simulink model "Metal_hydride_tank_Model_charge_Keow"  (R2022b)
settings: Solver=FixedStepAuto  StartTime=0.0  StopTime=54000  FixedStep=5e-3  MaxStep=0.005  RelTol=1e-3
values from neighbouring files (symbols this model uses):
  a = 13.7    [Metal_hydride_tank_Model_charge_Keow_run.m]
  A_s = 1.347    [Metal_hydride_tank_Model_charge_Keow_run.m]
  b = 3704    [Metal_hydride_tank_Model_charge_Keow_run.m]
  beta = 0.11414    [Metal_hydride_tank_Model_charge_Keow_run.m]
  C_a = 59.187    [Metal_hydride_tank_Model_charge_Keow_run.m]
  C_d = 9.57    [Metal_hydride_tank_Model_charge_Keow_run.m]
  C_pg = 14890    [Metal_hydride_tank_Model_charge_Keow_run.m]
  C_ps = 419    [Metal_hydride_tank_Model_charge_Keow_run.m]
  C_pw = 1860    [Metal_hydride_tank_Model_charge_Keow_run.m]
  Delta_Ha = 30478    [Metal_hydride_tank_Model_charge_Keow_run.m]
  Delta_Hd = 30800    [Metal_hydride_tank_Model_charge_Keow_run.m]
  E_a = 21179.6    [Metal_hydride_tank_Model_charge_Keow_run.m]
  E_d = 16420    [Metal_hydride_tank_Model_charge_Keow_run.m]
  epsilon = 0.5    [Metal_hydride_tank_Model_charge_Keow_run.m]
  f_w = 0.1667    [Metal_hydride_tank_Model_charge_Keow_run.m]
  m_MH = 47    [Metal_hydride_tank_Model_charge_Keow_run.m]
  MW_H2 = 2.01598e-3    (= 0.00201598)    [Metal_hydride_tank_Model_charge_Keow_run.m]
  P_0 = 101325    [Metal_hydride_tank_Model_charge_Keow_run.m]
  P_ref = 1500000    [Metal_hydride_tank_Model_charge_Keow_run.m]
  Phi = 0.33    [Metal_hydride_tank_Model_charge_Keow_run.m]
  Phi_0 = 0.008584    [Metal_hydride_tank_Model_charge_Keow_run.m]
  R_u = 8.314472    [Metal_hydride_tank_Model_charge_Keow_run.m]
  rho_H2 = 0.0897    [Metal_hydride_tank_Model_charge_Keow_run.m]
  rho_s0 = 8400    [Metal_hydride_tank_Model_charge_Keow_run.m]
  T_win = 293.15    [Metal_hydride_tank_Model_charge_Keow_run.m]
  U = 25    [Metal_hydride_tank_Model_charge_Keow_run.m]
  V_H2 = 7.849    [Metal_hydride_tank_Model_charge_Keow_run.m]
  V_tank = 0.0165    [Metal_hydride_tank_Model_charge_Keow_run.m]
settings Model: Creator=76593  LastModifiedBy=cmingrui
settings SolverCC: AlgebraicLoopSolver=TrustRegion
settings DataIOCC: ReturnWorkspaceOutputs=off
settings DebuggingCC: UnconnectedInputMsg=warning  UnconnectedOutputMsg=warning  UnconnectedLineMsg=warning  SFMachineParentedDataDiag=warning
settings ModelReferenceCC: EnableRefExpFcnMdlSchedulingChecks=on
settings RTWCC: DLArmComputeVersion=19.05

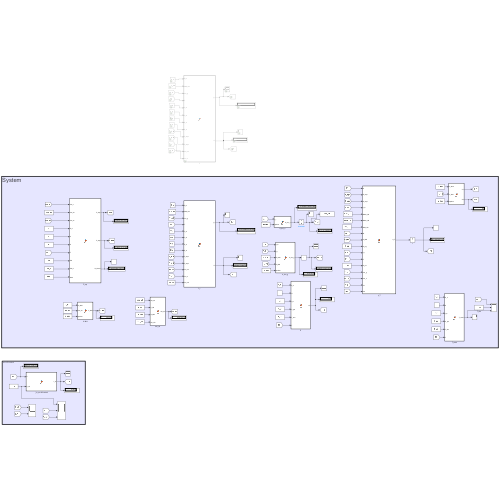
[thumbnail: Simulink's stored preview of the top-level diagram]
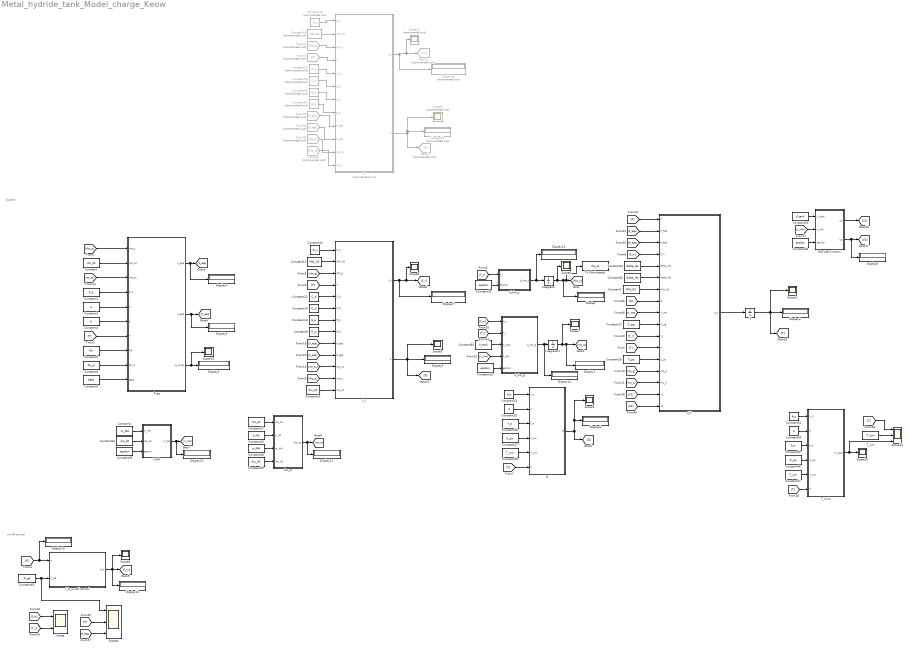
== system Metal_hydride_tank_Model_charge_Keow ==
  note: on-off control
  note: System
  1 : MATLAB Function  Commented=on  TreatAsAtomicUnit=on
  Constant{,24,31,37} (4 alike) : Constant  Value=rho_s0
  Constant1 : Constant  Value=m_MH
  Constant10 : Constant  Value=R_u
  Constant11 : Constant  Value=MW_H2
  Constant12 : Constant  Value=C_a
  Constant13 : Constant  Value=E_a
  Constant14 : Constant  Value=C_d
  Constant15 : Constant  Commented=on  Value=R_u
  Constant16 : Constant  Commented=on  Value=MW_H2
  Constant17 : Constant  Value=C_pg
  Constant{18..19,35..36} (4 alike) : Constant  Value=epsilon
  Constant2 : Constant  Value=P_0
  Constant20 : Constant  Value=C_ps
  Constant21 : Constant  Value=Delta_Ha
  Constant22 : Constant  Commented=on  Value=C_a
  Constant23 : Constant  Value=A_s
  Constant25 : Constant  Value=U
  Constant26 : Constant  Value=f_w
  Constant27 : Constant  Value=C_pw
  Constant28 : Constant  Value=T_win
  Constant29 : Constant  Value=V_tank
  Constant3 : Constant  Value=a
  Constant30 : Constant  Value=V_tank
  Constant32 : Constant  Value=Delta_Hd
  Constant33 : Constant  Commented=on  Value=E_a
  Constant34 : Constant  Commented=on  Value=C_d
  Constant38 : Constant  Value=m_MH
  Constant39 : Constant  Value=rho_H2
  Constant4 : Constant  Value=b
  Constant41 : Constant  Commented=on  Value=E_d
  Constant43 : Constant  Value=V_H2
  Constant47 : Constant  Value=T_win
  Constant48 : Constant  Value=C_pw
  Constant49 : Constant  Value=f_w
  Constant5 : Constant  Value=Phi
  Constant50 : Constant  Value=U
  Constant51 : Constant  Value=A_s
  Constant6 : Constant  Value=Phi_0
  Constant65 : Constant  Value=P_ref
  Constant7 : Constant  Value=MW_H2
  Constant8 : Constant  Value=E_d
  Constant9 : Constant  Value=beta
  Display{,1..14,19} (16 alike) : Display
  Display15 : Display  Commented=on
  Display16 : Display  Commented=on
  From26 : From  Commented=on  GotoTag=rho_ss
  From29 : From  Commented=on  GotoTag=P_eqa
  From30 : From  Commented=on  GotoTag=P_eqd
  From31 : From  Commented=on  GotoTag=rho_g
  From32 : From  Commented=on  GotoTag=rho_s
  From33 : From  Commented=on  GotoTag=T
  Goto11 : Goto  Commented=on  GotoTag=f_r
  Goto5 : Goto  Commented=on  GotoTag=P
  Integrator : Integrator  InitialCondition=8412.4
  Integrator1 : Integrator  InitialCondition=0.0831
  MATLAB Function : MATLAB Function  TreatAsAtomicUnit=on
  P_eq : MATLAB Function  TreatAsAtomicUnit=on
  Q : MATLAB Function  TreatAsAtomicUnit=on
  Scope : Scope  NumInputPorts=2
  Scope{1..3,6..10,15} (9 alike) : Scope
  Scope11 : Scope  NumInputPorts=3
  Scope12 : Scope  Commented=on
  Scope4 : Scope  NumInputPorts=3
  Scope5 : Scope  Commented=on
  T : Integrator  InitialCondition=293.15
  T_win : Constant  Value=T_win
  T_wout : MATLAB Function  TreatAsAtomicUnit=on
  To Workspace1 : ToWorkspace  VariableName=rho_s1  SampleTime=-1
  V_MH : MATLAB Function  TreatAsAtomicUnit=on
  d_T : MATLAB Function  TreatAsAtomicUnit=on
  d_rho_g : MATLAB Function  TreatAsAtomicUnit=on
  d_rho_s : MATLAB Function  TreatAsAtomicUnit=on
  f_in_on-off control : MATLAB Function  TreatAsAtomicUnit=on
  f_r : MATLAB Function  TreatAsAtomicUnit=on
  rho_ss : MATLAB Function  TreatAsAtomicUnit=on
  wires:
  Integrator/1 -> Scope6/1, Display/1, To Workspace1/1, [rho_s]
  d_rho_g/1(d_rho_g) -> Display14/1, Integrator1/1
  Integrator1/1 -> Scope7/1, Display1/1, [rho_g]
  d_T/1(d_T) -> T/1
  [T] -> d_T/12(T)
  [rho_s] -> P_eq/1(rho_s)
  Constant/1 -> P_eq/2(rho_s0)
  [rho_ss] -> P_eq/3(rho_ss)
  Constant2/1 -> P_eq/4(P_0)
  Constant3/1 -> P_eq/5(a)
  Constant4/1 -> P_eq/6(b)
  [T] -> P_eq/7(T)
  Constant5/1 -> P_eq/8(Phi)
  Constant6/1 -> P_eq/9(Phi_0)
  Constant9/1 -> P_eq/10(beta)
  Constant10/1 -> f_r/1(R_u)
  [T] -> f_r/4(T)
  Constant12/1 -> f_r/5(C_a)
  Constant13/1 -> f_r/7(E_a)
  [rho_ss] -> f_r/11(rho_ss)
  Constant17/1 -> d_T/10(C_pg)
  Constant19/1 -> d_rho_g/5(epsilon)
  Constant20/1 -> d_T/13(C_ps)
  Q/1(Q) -> [Q], Scope1/1, Display6/1
  [T] -> Q/6(T)
  Constant23/1 -> Q/1(A_s)
  Constant25/1 -> Q/2(U)
  Constant26/1 -> Q/3(f_w)
  Constant27/1 -> Q/4(C_pw)
  Constant28/1 -> Q/5(T_win)
  Constant30/1 -> d_rho_g/3(V_tank)
  [V_MH] -> d_rho_g/4(V_MH)
  f_r/2(P) -> Scope3/1, Display3/1, [P]
  Constant35/1 -> d_rho_s/2(epsilon)
  T/1 -> [T], Scope2/1, Display2/1
  P_eq/3(H_Hmax) -> Scope15/1, Display5/1
  [f_in] -> d_T/4(f_in)
  [rho_g] -> d_T/14(rho_g)
  [rho_s] -> d_T/15(rho_s)
  [f_in] -> d_rho_g/1(f_in)
  [f_r] -> d_rho_g/2(f_r)
  V_MH/1(V_MH) -> Display10/1, [V_MH]
  Constant24/1 -> V_MH/2(rho_s0)
  Constant36/1 -> V_MH/3(epsilon)
  Constant37/1 -> rho_ss/1(rho_s0)
  rho_ss/1(rho_ss) -> Display11/1, [rho_ss]
  Constant43/1 -> rho_ss/2(V_H2)
  Constant38/1 -> rho_ss/3(m_MH)
  Constant39/1 -> rho_ss/4(rho_H2)
  Constant1/1 -> V_MH/1(m_MH)
  Constant7/1 -> d_T/7(MW_H2)
  Constant8/1 -> f_r/8(E_d)
  Constant14/1 -> f_r/6(C_d)
  Constant31/1 -> f_r/13(rho_s0)
  P_eq/1(P_eqa) -> Display4/1, [P_eqa]
  P_eq/2(P_eqd) -> Display9/1, [P_eqd]
  [P_eqa] -> f_r/9(P_eqa)
  [P_eqd] -> f_r/10(P_eqd)
  [f_r] -> d_T/11(f_r)
  Constant21/1 -> d_T/5(Delta_Ha)
  Constant32/1 -> d_T/6(Delta_Hd)
  [P] -> d_T/1(P)
  [P_eqa] -> d_T/2(P_eqa)
  [rho_s] -> f_r/12(rho_s)
  [rho_g] -> f_r/3(rho_g)
  [P] -> Display19/1, f_in_on-off control/1(P)
  f_in_on-off control/1(f_in) -> Scope8/1, [f_in], Display12/1
  [f_in] -> Scope/1
  [f_r] -> Scope/2
  [P] -> Scope4/2
  Constant65/1 -> f_in_on-off control/2(P_ref), Scope4/1
  [P_eqa] -> Scope4/3
  [T] -> T_wout/6(T)
  Constant47/1 -> T_wout/5(T_win)
  Constant48/1 -> T_wout/4(C_pw)
  Constant49/1 -> T_wout/3(f_w)
  Constant50/1 -> T_wout/2(U)
  Constant51/1 -> T_wout/1(A_s)
  T_wout/1(T_wout) -> Scope11/3, Scope10/1
  [P_eqd] -> d_T/3(P_eqd)
  T_win/1 -> Scope11/2
  d_rho_s/1(d_rho_s) -> Integrator/1, Display13/1
  f_r/1(f_r) -> Display7/1, Scope9/1, [f_r]
  [f_r] -> d_rho_s/1(f_r)
  Constant11/1 -> f_r/2(MW_H2)
  [Q] -> d_T/8(Q)
  [V_MH] -> d_T/9(V_MH)
  MATLAB Function/1(V1) -> [V1]
  MATLAB Function/2(V2) -> Display8/1, [V2]
  Constant29/1 -> MATLAB Function/1(V_tank)
  [V_MH] -> MATLAB Function/2(V_MH)
  Constant18/1 -> MATLAB Function/3(epsilon)
  [T] -> Scope11/1
  [V1] -> d_T/16(V1)
  [V2] -> d_T/17(V2)
  Constant16/1 -> 1/2(MW_H2)
  1/1(f_r) -> Goto11/1, Scope12/1, Display16/1
  From31/1 -> 1/3(rho_g)
  From32/1 -> 1/12(rho_s)
  From30/1 -> 1/10(P_eqd)
  From29/1 -> 1/9(P_eqa)
  Constant34/1 -> 1/6(C_d)
  Constant41/1 -> 1/8(E_d)
  1/2(P) -> Display15/1, Scope5/1, Goto5/1
  From26/1 -> 1/11(rho_ss)
  Constant33/1 -> 1/7(E_a)
  Constant22/1 -> 1/5(C_a)
  From33/1 -> 1/4(T)
  Constant15/1 -> 1/1(R_u)

== matlab function Metal_hydride_tank_Model_charge_Keow/d_rho_g ==
  data: f_in input; f_r input; V_tank input; V_MH input; d_rho_g output; epsilon input
function d_rho_g = fcn(f_in,f_r,V_tank,V_MH,epsilon)

V1=V_tank/V_MH-1+epsilon;
d_rho_g = (f_in-f_r)/V1;

== matlab function Metal_hydride_tank_Model_charge_Keow/d_T ==
  data: P input; P_eqa input; P_eqd input; f_in input; Delta_Ha input; Delta_Hd input; MW_H2 input; Q input; V_MH input; C_pg input; d_T output; f_r input; T input; C_ps input; rho_g input; rho_s input; V1 input; V2 input
 function d_T  = fcn(P,P_eqa,P_eqd,f_in,Delta_Ha,Delta_Hd,MW_H2,Q,V_MH,C_pg,f_r,T,C_ps,rho_g,rho_s,V1,V2)

if P>P_eqa
    d_T = (-C_pg*(f_in-f_r)*T-C_ps*f_r*T+f_r*Delta_Ha/MW_H2+Q/V_MH)/(V1*C_pg*rho_g+V2*C_ps*rho_s);
elseif P<P_eqd
    d_T = (-C_pg*(f_in-f_r)*T-C_ps*f_r*T+f_r*Delta_Hd/MW_H2+Q/V_MH)/(V1*C_pg*rho_g+V2*C_ps*rho_s);
else
    d_T = (-C_pg*f_in*T+Q/V_MH)/(V1*C_pg*rho_g+V2*C_ps*rho_s);
end

== matlab function Metal_hydride_tank_Model_charge_Keow/Q ==
  data: A_s input; U input; f_w input; Q output; C_pw input; T_win input; T input
function Q = fcn(A_s,U,f_w,C_pw,T_win,T)

alpha=U*A_s/(f_w*C_pw);
Q = f_w*C_pw*(T_win-T)*(1-exp(-alpha));

== matlab function Metal_hydride_tank_Model_charge_Keow/V_MH ==
  data: m_MH input; rho_s0 input; V_MH output; epsilon input
function V_MH = fcn(m_MH,rho_s0,epsilon)

V_MH = m_MH/(rho_s0*epsilon);

== matlab function Metal_hydride_tank_Model_charge_Keow/rho_ss ==
  data: rho_s0 input; rho_ss output; V_H2 input; m_MH input; rho_H2 input
function rho_ss = fcn(rho_s0,V_H2,m_MH,rho_H2)

rho_ss = rho_s0*(1+V_H2/m_MH*rho_H2);

== matlab function Metal_hydride_tank_Model_charge_Keow/f_in_on-off control ==
  data: P input; f_in output; P_ref input
function f_in = fcn(P,P_ref)

if P<P_ref
   f_in=0.0012;
else
   f_in=0;
end

== matlab function Metal_hydride_tank_Model_charge_Keow/T_wout ==
  data: A_s input; U input; f_w input; T_wout output; C_pw input; T_win input; T input
function T_wout = fcn(A_s,U,f_w,C_pw,T_win,T)

alpha=U*A_s/(f_w*C_pw);
T_wout = T+(T_win-T)*exp(-alpha);

== matlab function Metal_hydride_tank_Model_charge_Keow/MATLAB Function ==
  data: V_tank input; V1 output; V_MH input; epsilon input; V2 output
function [V1,V2] = fcn(V_tank,V_MH,epsilon)

V1=V_tank/V_MH-1+epsilon;
V2=1-epsilon;

== matlab function Metal_hydride_tank_Model_charge_Keow/f_r ==
  data: R_u input; MW_H2 input; rho_g input; T input; C_a input; C_d input; E_a input; E_d input; P_eqa input; P_eqd input; rho_ss input; rho_s input; f_r output; rho_s0 input; P output
function [f_r,P] = fcn(R_u,MW_H2,rho_g,T,C_a,C_d,E_a,E_d,P_eqa,P_eqd,rho_ss,rho_s,rho_s0)

P=rho_g*R_u/MW_H2*T;
if P>P_eqa
    f_r = C_a*exp(-E_a/(R_u*T))*log(P/P_eqa)*(rho_ss-rho_s);
elseif P<P_eqd
    f_r = C_d*exp(-E_d/(R_u*T))*((P-P_eqd)/P_eqd)*(rho_s-rho_s0);
else
    f_r=0;
end

== matlab function Metal_hydride_tank_Model_charge_Keow/P_eq ==
  data: rho_s input; P_eqa output; P_eqd output; rho_s0 input; rho_ss input; P_0 input; a input; b input; T input; Phi input; Phi_0 input; beta input; H_Hmax output
function [P_eqa,P_eqd,H_Hmax]  = fcn(rho_s,rho_s0,rho_ss,P_0,a,b,T,Phi,Phi_0,beta)

H_Hmax=(rho_s-rho_s0)/(rho_ss-rho_s0);
P_eqa = P_0*exp(a-b/T+(Phi+Phi_0)*tan(pi*(H_Hmax-0.5))+beta/2);
P_eqd = P_0*exp(a-b/T+(Phi-Phi_0)*tan(pi*(H_Hmax-0.5))-beta/2);

== matlab function Metal_hydride_tank_Model_charge_Keow/d_rho_s ==
  data: f_r input; d_rho_s output; epsilon input
function d_rho_s = fcn(f_r,epsilon)

V2=1-epsilon;
d_rho_s = f_r/V2;

== matlab function Metal_hydride_tank_Model_charge_Keow/1 ==
  data: R_u input; MW_H2 input; rho_g input; T input; C_a input; C_d input; E_a input; E_d input; P_eqa input; P_eqd input; rho_ss input; rho_s input; f_r output; P output
function [f_r,P] = fcn(R_u,MW_H2,rho_g,T,C_a,C_d,E_a,E_d,P_eqa,P_eqd,rho_ss,rho_s)

P=rho_g*R_u/MW_H2*T;
if P>P_eqa
    f_r = C_a*exp(-E_a/(R_u*T))*log(P/P_eqa)*(rho_ss-rho_s);
elseif P<P_eqd
    f_r = C_d*exp(-E_d/(R_u*T))*((P-P_eqd)/P_eqd)*rho_s;
else
    f_r=0;
end
